simulink model "test_mex"  (R2016b)
settings: Solver=FixedStepAuto  StartTime=0.0  StopTime=0.5  FixedStep=0.50  RelTol=1e-3
settings Model: Creator=jreher  LastModifiedBy=jreher
settings RTWCC: SystemTargetFile=sldrt.tlc  TemplateMakefile=sldrt.tmf  Description=Simulink Desktop Real-Time  RTWCompilerOptimization=on
settings CodeAppCC: MaxIdLength=95
settings SimulinkDesktopRealTimeCC: TargetPreCompLibLocation=D:\Program Files\MATLAB\R2016b\toolbox\sldrt\lib\win64  SupportVariableSizeSignals=off

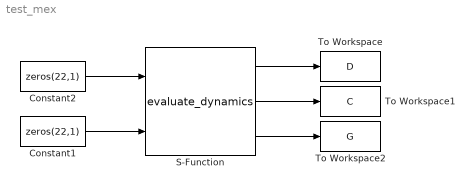
== system test_mex ==
  Constant1 : Constant  Value=zeros(22,1)
  Constant2 : Constant  Value=zeros(22,1)
  S-Function : S-Function  FunctionName=evaluate_dynamics  SFunctionDeploymentMode=off  EnableBusSupport=off
  To Workspace : ToWorkspace  VariableName=D  SaveFormat=Timeseries  SampleTime=-1
  To Workspace1 : ToWorkspace  VariableName=C  SaveFormat=Timeseries  SampleTime=-1
  To Workspace2 : ToWorkspace  VariableName=G  SaveFormat=Timeseries  SampleTime=-1
  wires:
  Constant1/1 -> S-Function/2
  S-Function/1 -> To Workspace/1
  S-Function/2 -> To Workspace1/1
  S-Function/3 -> To Workspace2/1
  Constant2/1 -> S-Function/1
